simulink model "comparando_bloco_inversor"  (R2012b)
settings: Solver=ode45  StartTime=0.0  StopTime=60  RelTol=1e-3
undefined symbols (not defined in the file): Vcc
libraries: simulink x12
settings Model: Creator=Juliano  LastModifiedBy=Juliano

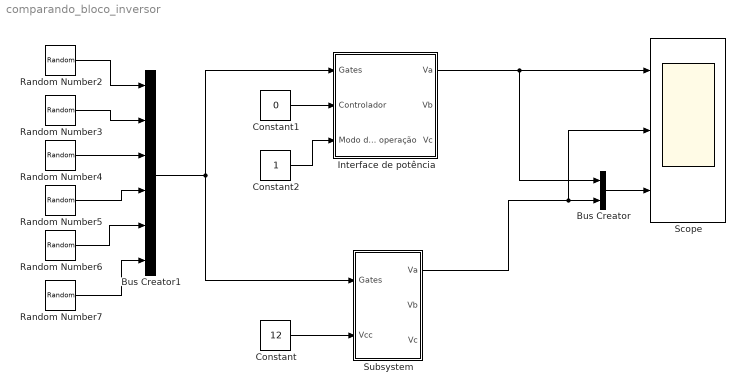
== system comparando_bloco_inversor ==
  Bus Creator : BusCreator  Inputs=2
  Bus Creator1 : BusCreator  Inputs=6
  Constant : Constant  Value=12
  Constant1 : Constant  Value=0
  Constant2 : Constant
  Interface de potência : Subsystem
  Random Number2 : RandomNumber  Variance=20  SampleTime=0.1
  Random Number3 : RandomNumber  Variance=20  Seed=1  SampleTime=0.1
  Random Number4 : RandomNumber  Variance=20  Seed=2  SampleTime=0.1
  Random Number5 : RandomNumber  Variance=20  Seed=3  SampleTime=0.1
  Random Number6 : RandomNumber  Variance=20  Seed=4  SampleTime=0.1
  Random Number7 : RandomNumber  Variance=20  Seed=5  SampleTime=0.1
  Scope : Scope  NumInputPorts=3
      settings: TimeRange=0.5  YMin=0~0~0  YMax=800000~800000~800000
  Subsystem : Subsystem
  wires:
  Bus Creator/1 -> Scope/3
  Interface de potência/1(Va) -> Bus Creator/1, Scope/1
  Subsystem/1(Va) -> Scope/2, Bus Creator/2
  Constant/1 -> Subsystem/2(Vcc)
  Constant1/1 -> Interface de potência/2(Controlador)
  Constant2/1 -> Interface de potência/3(Modo de operação)
  Random Number2/1 -> Bus Creator1/1
  Random Number3/1 -> Bus Creator1/2
  Random Number4/1 -> Bus Creator1/3
  Random Number5/1 -> Bus Creator1/4
  Random Number7/1 -> Bus Creator1/6
  Random Number6/1 -> Bus Creator1/5
  Bus Creator1/1 -> Subsystem/1(Gates), Interface de potência/1(Gates)

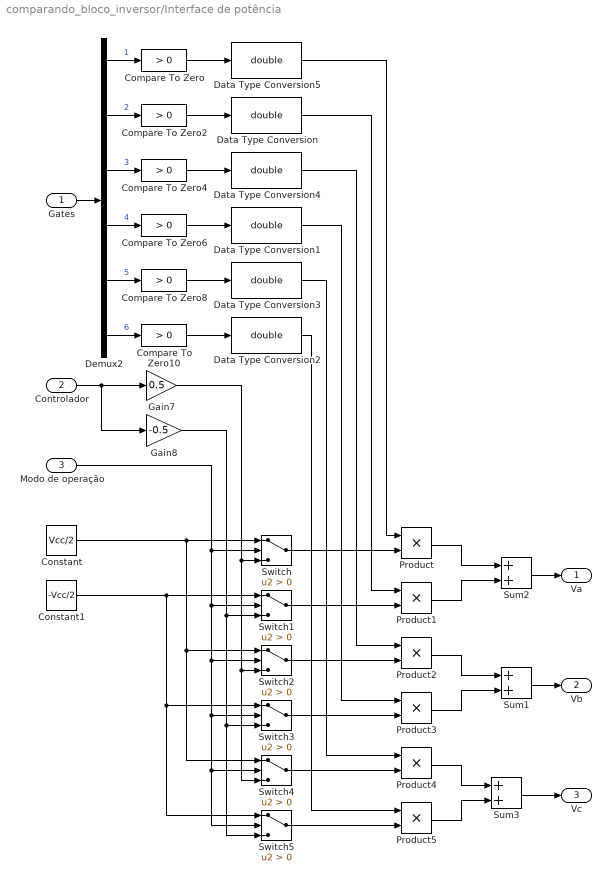
== system comparando_bloco_inversor/Interface de potência ==
  Gates : Inport
  Controlador : Inport  Port=2
  Modo de operação : Inport  Port=3
  Compare To Zero : simulink/Logic and Bit Operations/Compare To Zero  relop=>  OutDataTypeStr=uint8  ZeroCross=off
  Compare To Zero{2,6,8,10} (4 alike) : simulink/Logic and Bit Operations/Compare To Zero  relop=>  OutDataTypeStr=boolean  ZeroCross=off
  Compare To Zero4 : simulink/Logic and Bit Operations/Compare To Zero  relop=>  OutDataTypeStr=uint8  ZeroCross=off
  Constant : Constant  Value=Vcc/2
  Constant1 : Constant  Value=-Vcc/2
  Data Type Conversion{,1..5} (6 alike) : DataTypeConversion  OutDataTypeStr=double
  Demux2 : Demux  Outputs=6
  Gain7 : Gain  Gain=0.5
  Gain8 : Gain  Gain=-0.5
  Product{,1..5} (6 alike) : Product  RndMeth=Zero
  Sum1 : Sum  SaturateOnIntegerOverflow=on
  Sum2 : Sum  SaturateOnIntegerOverflow=on
  Sum3 : Sum  SaturateOnIntegerOverflow=on
  Switch{,1..5} (6 alike) : Switch  Criteria=u2 > Threshold
  Va : Outport
  Vb : Outport  Port=2
  Vc : Outport  Port=3
  wires:
  Data Type Conversion5/1 -> Product/1
  Data Type Conversion/1 -> Product1/1
  Data Type Conversion4/1 -> Product2/1
  Data Type Conversion1/1 -> Product3/1
  Data Type Conversion3/1 -> Product4/1
  Data Type Conversion2/1 -> Product5/1
  Product5/1 -> Sum3/2
  Product4/1 -> Sum3/1
  Product3/1 -> Sum1/2
  Product2/1 -> Sum1/1
  Product1/1 -> Sum2/2
  Product/1 -> Sum2/1
  Switch5/1 -> Product5/2
  Switch4/1 -> Product4/2
  Switch3/1 -> Product3/2
  Switch2/1 -> Product2/2
  Switch1/1 -> Product1/2
  Switch/1 -> Product/2
  Compare To Zero10/1 -> Data Type Conversion2/1
  Compare To Zero8/1 -> Data Type Conversion3/1
  Compare To Zero6/1 -> Data Type Conversion1/1
  Compare To Zero4/1 -> Data Type Conversion4/1
  Compare To Zero2/1 -> Data Type Conversion/1
  Compare To Zero/1 -> Data Type Conversion5/1
  Demux2/6 -> Compare To Zero10/1  "6"
  Demux2/5 -> Compare To Zero8/1  "5"
  Demux2/4 -> Compare To Zero6/1  "4"
  Demux2/3 -> Compare To Zero4/1  "3"
  Demux2/2 -> Compare To Zero2/1  "2"
  Demux2/1 -> Compare To Zero/1  "1"
  Gates/1 -> Demux2/1
  Modo de operação/1 -> Switch5/2, Switch4/2, Switch3/2, Switch2/2, Switch1/2, Switch/2
  Gain8/1 -> Switch5/3, Switch3/3, Switch1/3
  Gain7/1 -> Switch4/3, Switch2/3, Switch/3
  Controlador/1 -> Gain8/1, Gain7/1
  Constant1/1 -> Switch5/1, Switch3/1, Switch1/1
  Constant/1 -> Switch4/1, Switch2/1, Switch/1
  Sum2/1 -> Va/1
  Sum3/1 -> Vc/1
  Sum1/1 -> Vb/1

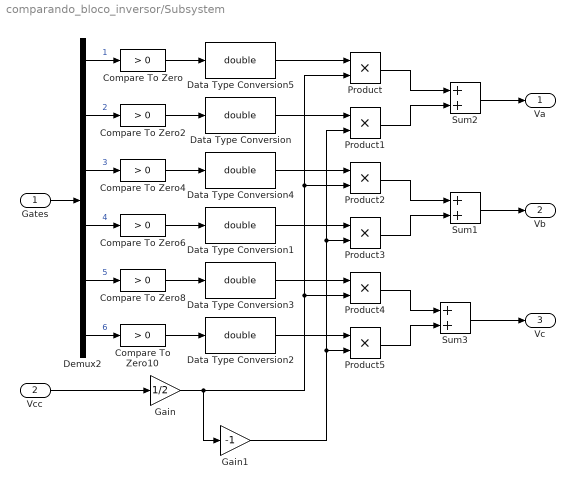
== system comparando_bloco_inversor/Subsystem ==
  Gates : Inport
  Vcc : Inport  Port=2
  Compare To Zero : simulink/Logic and Bit Operations/Compare To Zero  relop=>  OutDataTypeStr=uint8  ZeroCross=off
  Compare To Zero{2,6,8,10} (4 alike) : simulink/Logic and Bit Operations/Compare To Zero  relop=>  OutDataTypeStr=boolean  ZeroCross=off
  Compare To Zero4 : simulink/Logic and Bit Operations/Compare To Zero  relop=>  OutDataTypeStr=uint8  ZeroCross=off
  Data Type Conversion{,1..5} (6 alike) : DataTypeConversion  OutDataTypeStr=double
  Demux2 : Demux  Outputs=6
  Gain : Gain  Gain=1/2
  Gain1 : Gain  Gain=-1
  Product{,1..5} (6 alike) : Product  RndMeth=Zero
  Sum1 : Sum  SaturateOnIntegerOverflow=on
  Sum2 : Sum  SaturateOnIntegerOverflow=on
  Sum3 : Sum  SaturateOnIntegerOverflow=on
  Va : Outport
  Vb : Outport  Port=2
  Vc : Outport  Port=3
  wires:
  Gain/1 -> Product/2, Product2/2, Product4/2, Gain1/1
  Gain1/1 -> Product1/2, Product3/2, Product5/2
  Data Type Conversion5/1 -> Product/1
  Data Type Conversion/1 -> Product1/1
  Data Type Conversion4/1 -> Product2/1
  Data Type Conversion1/1 -> Product3/1
  Data Type Conversion3/1 -> Product4/1
  Data Type Conversion2/1 -> Product5/1
  Product5/1 -> Sum3/2
  Product4/1 -> Sum3/1
  Product3/1 -> Sum1/2
  Product2/1 -> Sum1/1
  Product1/1 -> Sum2/2
  Product/1 -> Sum2/1
  Compare To Zero10/1 -> Data Type Conversion2/1
  Compare To Zero8/1 -> Data Type Conversion3/1
  Compare To Zero6/1 -> Data Type Conversion1/1
  Compare To Zero4/1 -> Data Type Conversion4/1
  Compare To Zero2/1 -> Data Type Conversion/1
  Compare To Zero/1 -> Data Type Conversion5/1
  Demux2/6 -> Compare To Zero10/1  "6"
  Demux2/5 -> Compare To Zero8/1  "5"
  Demux2/4 -> Compare To Zero6/1  "4"
  Demux2/3 -> Compare To Zero4/1  "3"
  Demux2/2 -> Compare To Zero2/1  "2"
  Demux2/1 -> Compare To Zero/1  "1"
  Gates/1 -> Demux2/1
  Sum2/1 -> Va/1
  Sum3/1 -> Vc/1
  Sum1/1 -> Vb/1
  Vcc/1 -> Gain/1
